simulink model "ClosedLoop_CqCscCi"  (R2022b)
settings: Solver=VariableStepAuto  StartTime=0.0  StopTime=10.0  RelTol=1e-3
libraries: cstblocks x5
settings Model: Creator=antoninrenoir  LastModifiedBy=emili

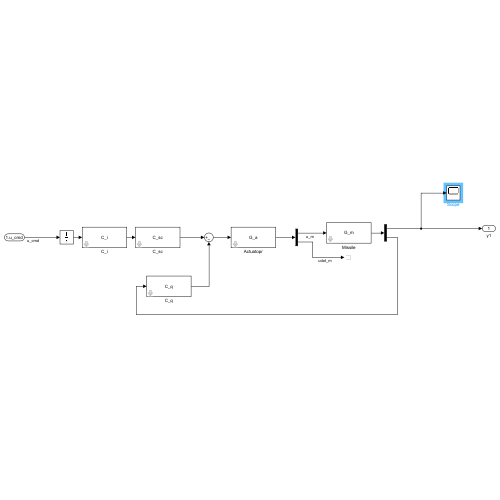
[thumbnail: Simulink's stored preview of the top-level diagram]
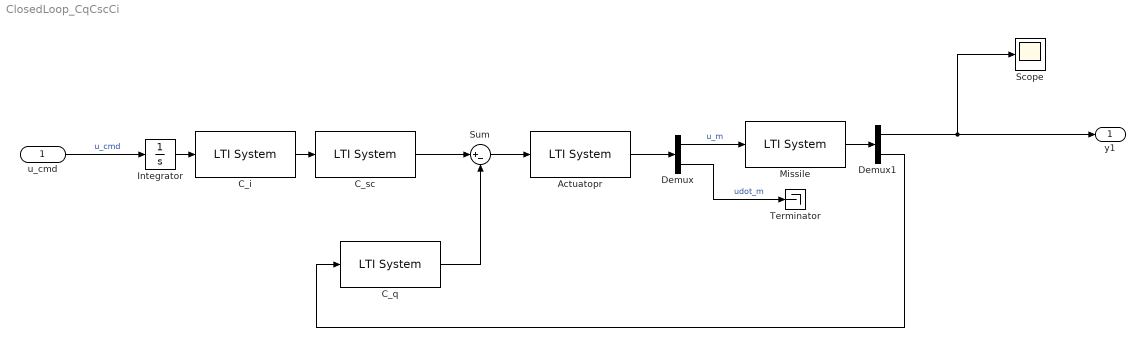
== system ClosedLoop_CqCscCi ==
  u_cmd : Inport
  Actuatopr : cstblocks/LTI System  sys=G_a  IC=[]
  C_i : cstblocks/LTI System  sys=C_i  IC=[]
  C_q : cstblocks/LTI System  sys=C_q  IC=[]
  C_sc : cstblocks/LTI System  sys=C_sc  IC=[]
  Demux : Demux  Outputs=2
  Demux1 : Demux  Outputs=2
  Integrator : Integrator
  Missile : cstblocks/LTI System  sys=G_m  IC=[]
  Scope : Scope
  Sum : Sum  Inputs=|+-
  Terminator : Terminator
  y1 : Outport
  wires:
  C_sc/1 -> Sum/1
  Demux1/2 -> C_q/1
  Sum/1 -> Actuatopr/1
  Demux/1 -> Missile/1  "u_m"
  Missile/1 -> Demux1/1
  Demux1/1 -> Scope/1, y1/1
  u_cmd/1 -> Integrator/1  "u_cmd"
  Demux/2 -> Terminator/1  "udot_m"
  Actuatopr/1 -> Demux/1
  C_q/1 -> Sum/2
  C_i/1 -> C_sc/1
  Integrator/1 -> C_i/1
